simulink model "Target_Control_System"  (R2021b)
settings: Solver=FixedStepDiscrete  StartTime=0.0  StopTime=5  RelTol=1e-3
PreLoadFcn:
  | RTWConfigurationCB('preloadfcn', bdroot);
PostLoadFcn:
  | load('configuration/data_struct.mat');
  | load('configuration/fluxMaps_propMotor.mat');
  | load('configuration/parameterInit_PROP.mat');
  | load('configuration/parameterInit_PUMP.mat');
  | load('configuration/parameterInit_PITCH.mat');
  | load('configuration/parameterInit_TILT.mat');
  | %load('configuration/base_workspace_signal_definition.mat');
  | %load('resolvedatastores_to_baseworkspace_for_faster_simulation.mat');
model workspace (MAT data in the model file):
  SIMULATION_OPTIONS : Simulink.Parameter (value not decoded)
  TARGET_CODE_GEN : Simulink.Parameter (value not decoded)
  TCS_SAMPLE_FREQ_HZ : Simulink.Parameter (value not decoded)
symbols that are objects in the model workspace (value not decoded): TARGET_CODE_GEN, TCS_SAMPLE_FREQ_HZ
undefined symbols (not defined in the file): A_DQ_REF_LPF_INIT__PITCH, A_DQ_REF_LPF_INIT__PROP, A_DQ_REF_LPF_INIT__PUMP, A_DQ_REF_LPF_INIT__TILT, A_OBSERVER_CONFIDENCE_INIT__PITCH, A_OBSERVER_CONFIDENCE_INIT__PROP, A_OBSERVER_CONFIDENCE_INIT__PUMP, A_OBSERVER_CONFIDENCE_INIT__TILT, ACTUATOR_MAX_ANGLE_TRIP__PITCH, ACTUATOR_MIN_ANGLE_TRIP__PITCH, ACTUATOR_POS_SENSOR_INV_DIRECTION__PITCH, ACTUATOR_POS_SENSOR_INV_DIRECTION__TILT, ACTUATOR_POS_SENSOR_OFFSET__PITCH, ACTUATOR_POS_SENSOR_OFFSET__TILT, ADC_scaler1_baseaddr_TILT, ADC_SCALER_FLOAT_TO_FIXPOINT_EXPANSION, ANGLE_ELEC_FROM_SENSOR_OFFSET_INIT__PITCH, ANGLE_ELEC_FROM_SENSOR_OFFSET_INIT__PROP, ANGLE_ELEC_FROM_SENSOR_OFFSET_INIT__PUMP, ANGLE_ELEC_FROM_SENSOR_OFFSET_INIT__TILT, AUTO_CLEAR_FAULTS_ENABLED__PITCH, AUTO_CLEAR_FAULTS_ENABLED__PROP, AUTO_CLEAR_FAULTS_ENABLED__PUMP, AUTO_CLEAR_FAULTS_ENABLED__TILT, AUTO_CLEAR_FAULTS_WAIT_TICKS__PITCH, AUTO_CLEAR_FAULTS_WAIT_TICKS__PROP, AUTO_CLEAR_FAULTS_WAIT_TICKS__PUMP, AUTO_CLEAR_FAULTS_WAIT_TICKS__TILT, AUTO_I_ZERO_IDLE_TICKS__PITCH, AUTO_I_ZERO_IDLE_TICKS__PROP, AUTO_I_ZERO_IDLE_TICKS__PUMP, AUTO_I_ZERO_IDLE_TICKS__TILT, AUTO_I_ZERO_OFFSET_IDC_THRESHOLD__PITCH, AUTO_I_ZERO_OFFSET_IDC_THRESHOLD__PROP, AUTO_I_ZERO_OFFSET_IDC_THRESHOLD__PUMP, AUTO_I_ZERO_OFFSET_IDC_THRESHOLD__TILT, AUTO_I_ZERO_OFFSET_IPH_THRESHOLD__PITCH, AUTO_I_ZERO_OFFSET_IPH_THRESHOLD__PROP, AUTO_I_ZERO_OFFSET_IPH_THRESHOLD__PUMP, AUTO_I_ZERO_OFFSET_IPH_THRESHOLD__TILT, AUTO_SENSORLESS_SWITCHOVER_DISABLE_OMEGA, AUTO_SENSORLESS_SWITCHOVER_ENABLE_OMEGA, AUTO_SENSORLESS_SWITCHOVER_MIN_CONFIDENCE, AUXILIARY_PROTECTION_UNIT_BASEADDR__TILT, blanking_max_error_omega_INIT_PITCH, blanking_max_error_omega_INIT_TILT, blanking_max_error_position_INIT_PITCH, blanking_max_error_position_INIT_TILT, BRUTE_START_I_Q_REF_RAMP_SPEED__PITCH, BRUTE_START_I_Q_REF_RAMP_SPEED__PROP, BRUTE_START_I_Q_REF_RAMP_SPEED__PUMP, BRUTE_START_I_Q_REF_RAMP_SPEED__TILT, CONTROL_LOOP_DT_INIT__PITCH, CONTROL_LOOP_DT_INIT__PROP, CONTROL_LOOP_DT_INIT__PUMP, CONTROL_LOOP_DT_INIT__TILT, CORRECTION_FILTER_SCALE__PITCH, CORRECTION_FILTER_SCALE__PROP, CORRECTION_FILTER_SCALE__PUMP, CORRECTION_FILTER_SCALE__TILT ... (+458)
libraries: simulink x178, Reusables_Lib x24
(part 6 of 47)

== system Target_Control_System/Target_Control_System/InterruptFunction/pitchMotor_isrTask/abcToAlphaBeta ==
  abcToAlphaBeta : TriggerPort  TriggerType=function-call  VariantControl=Variant
  Alpha-Beta Calcs1 : Subsystem
  Calc Angle From Speed : Subsystem
  Constant1 : Constant  Value=TARGET_CODE_GEN  SampleTime=-1
  Data Store Read1 : DataStoreRead  DataStoreName=oPitch  DataStoreElements=oPitch.oIsr_.oState_.fUbPostlpf_  IndexOptions=Index vector (dialog)  Indices=1  OutputSizes=1
  Data Store Read13 : DataStoreRead  DataStoreName=oPitch  DataStoreElements=oPitch.oIsr_.oIn_.oAdcData_.fIa_  IndexOptions=Index vector (dialog)  Indices=1  OutputSizes=1
  Data Store Read14 : DataStoreRead  DataStoreName=oPitch  DataStoreElements=oPitch.oIsr_.oIn_.oAdcData_.fIb_  IndexOptions=Index vector (dialog)  Indices=1  OutputSizes=1
  Data Store Read15 : DataStoreRead  DataStoreName=oPitch  DataStoreElements=oPitch.oIsr_.oIn_.oAdcData_.fIc_  IndexOptions=Index vector (dialog)  Indices=1  OutputSizes=1
  Data Store Read16 : DataStoreRead  DataStoreName=oPitch  DataStoreElements=oPitch.oIsr_.oState_.fUaPostlpf_  IndexOptions=Index vector (dialog)  Indices=1  OutputSizes=1
  Data Store Read17 : DataStoreRead  DataStoreName=oPitch  DataStoreElements=oPitch.oIsr_.oState_.fUcPostlpf_  IndexOptions=Index vector (dialog)  Indices=1  OutputSizes=1
  Data Store Read2 : DataStoreRead  DataStoreName=oPitch  DataStoreElements=oPitch.oIsr_.oIn_.fUphFilterDelayAngleRad_  IndexOptions=Index vector (dialog)  Indices=1  OutputSizes=1
  Data Store Read4 : DataStoreRead  DataStoreName=oPitch  DataStoreElements=oPitch.oIsr_.oState_.fOmegaEObserverRaw2_  IndexOptions=Index vector (dialog)  Indices=1  OutputSizes=1
  Data Store Read8 : DataStoreRead  DataStoreName=oPitch  DataStoreElements=oPitch.oIsr_.oParam_.iInverseDirection_  IndexOptions=Index vector (dialog)  Indices=1  OutputSizes=1
  Data Store Write1 : DataStoreWrite  DataStoreName=oPitch  DataStoreElements=oPitch.oIsr_.oState_.fFluxMainAngleUltraRaw_  IndexOptions=Index vector (dialog)  Indices=1  OutputSizes=1
  Data Store Write2 : DataStoreWrite  DataStoreName=oPitch  DataStoreElements=oPitch.oIsr_.oState_.fIAlpha_  IndexOptions=Index vector (dialog)  Indices=1  OutputSizes=1
  Data Store Write3 : DataStoreWrite  DataStoreName=oPitch  DataStoreElements=oPitch.oIsr_.oState_.fIBeta_  IndexOptions=Index vector (dialog)  Indices=1  OutputSizes=1
  Data Store Write4 : DataStoreWrite  DataStoreName=oPitch  DataStoreElements=oPitch.oIsr_.oState_.fUAlpha_  IndexOptions=Index vector (dialog)  Indices=1  OutputSizes=1
  Data Store Write5 : DataStoreWrite  DataStoreName=oPitch  DataStoreElements=oPitch.oIsr_.oState_.fUBeta_  IndexOptions=Index vector (dialog)  Indices=1  OutputSizes=1
  ModelSource : Subsystem  Commented=on  Variant=on
  NOT1 : Logic  Operator=NOT  AllPortsSameDT=off  OutDataTypeStr=boolean
  vsincos()1 : Subsystem  TreatAsAtomicUnit=on
  wires:
  Data Store Read4/1 -> Calc Angle From Speed/1(Omega)
  NOT1/1 -> vsincos()1/Enable
  Alpha-Beta Calcs1/1(fIAlpha) -> Data Store Write2/1
  Data Store Read16/1 -> Alpha-Beta Calcs1/5(fUaPostlpf)
  Data Store Read8/1 -> Alpha-Beta Calcs1/1(iInverseDirection)
  Data Store Read1/1 -> Alpha-Beta Calcs1/6(fUbPostlpf)
  Alpha-Beta Calcs1/3(fUAlpha) -> Data Store Write4/1
  Data Store Read15/1 -> Alpha-Beta Calcs1/4(fIc)
  Alpha-Beta Calcs1/2(fIBeta) -> Data Store Write3/1
  Constant1/1 -> NOT1/1
  Data Store Read13/1 -> Alpha-Beta Calcs1/2(fIa)
  Data Store Read17/1 -> Alpha-Beta Calcs1/7(fUcPostlpf)
  Data Store Read14/1 -> Alpha-Beta Calcs1/3(fIb)
  Alpha-Beta Calcs1/4(fUBeta) -> Data Store Write5/1
  Calc Angle From Speed/1(fFluxMainAngleRaw2) -> vsincos()1/2(fFluxMainAngleRaw2), Data Store Write1/1
  Data Store Read2/1 -> vsincos()1/1(fUphFilterDelayAngleRad)

== system Target_Control_System/Target_Control_System/InterruptFunction/pitchMotor_isrTask/currentController ==
  currentController : TriggerPort  TriggerType=function-call  VariantControl=Variant
  Current Controller : Subsystem
  Data Store Read4 : DataStoreRead  DataStoreName=oPitch  DataStoreElements=oPitch.oIsr_.oIn_.uiCurrentControllerActive_  IndexOptions=Index vector (dialog)  Indices=1  OutputSizes=1
  wires:
  Data Store Read4/1 -> Current Controller/Enable

== system Target_Control_System/Target_Control_System/InterruptFunction/pitchMotor_isrTask/dqTransform ==
  dqTransform : TriggerPort  TriggerType=function-call  VariantControl=Variant
  DQ Transform : Subsystem
  Data Store Read1 : DataStoreRead  DataStoreName=oPitch  DataStoreElements=oPitch.oIsr_.oState_.fFluxMainMagnitudeLpf_  IndexOptions=Index vector (dialog)  Indices=1  OutputSizes=1
  Data Store Read2 : DataStoreRead  DataStoreName=oPitch  DataStoreElements=oPitch.oIsr_.oState_.fIBeta_  IndexOptions=Index vector (dialog)  Indices=1  OutputSizes=1
  Data Store Read3 : DataStoreRead  DataStoreName=oPitch  DataStoreElements=oPitch.oIsr_.oState_.fIq_  IndexOptions=Index vector (dialog)  Indices=1  OutputSizes=1
  Data Store Read4 : DataStoreRead  DataStoreName=oPitch  DataStoreElements=oPitch.oMot_.oParam_.fPolePairs_  IndexOptions=Index vector (dialog)  Indices=1  OutputSizes=1
  Data Store Read5 : DataStoreRead  DataStoreName=oPitch  DataStoreElements=oPitch.oIsr_.oState_.fIAlpha_  IndexOptions=Index vector (dialog)  Indices=1  OutputSizes=1
  Data Store Write1 : DataStoreWrite  DataStoreName=oPitch  DataStoreElements=oPitch.oIsr_.oOut_.fTEstimate_  IndexOptions=Index vector (dialog)  Indices=1  OutputSizes=1
  Data Store Write2 : DataStoreWrite  DataStoreName=oPitch  DataStoreElements=oPitch.oIsr_.oState_.fId_  IndexOptions=Index vector (dialog)  Indices=1  OutputSizes=1
  Data Store Write3 : DataStoreWrite  DataStoreName=oPitch  DataStoreElements=oPitch.oIsr_.oState_.fIq_  IndexOptions=Index vector (dialog)  Indices=1  OutputSizes=1
  Data Store Write4 : DataStoreWrite  DataStoreName=oPitch  DataStoreElements=oPitch.oIsr_.oOut_.fIPhaseMagnitude_  IndexOptions=Index vector (dialog)  Indices=1  OutputSizes=1
  Torque_Estimation_Pitch : Subsystem
  wires:
  DQ Transform/1(fId) -> Data Store Write2/1
  DQ Transform/3(fIPhaseMagnitude) -> Data Store Write4/1
  Data Store Read3/1 -> Torque_Estimation_Pitch/3(fIq)
  Torque_Estimation_Pitch/1(fTEstimate) -> Data Store Write1/1
  Data Store Read5/1 -> DQ Transform/1(fIAlpha)
  Data Store Read1/1 -> Torque_Estimation_Pitch/2(fFluxMainMagnitudeLpf)
  Data Store Read2/1 -> DQ Transform/2(fIBeta)
  Data Store Read4/1 -> Torque_Estimation_Pitch/1(fPolePairs)
  DQ Transform/2(fIq) -> Data Store Write3/1

== system Target_Control_System/Target_Control_System/InterruptFunction/pitchMotor_isrTask/fluxAngleCalculations ==
  fluxAngleCalculation : TriggerPort  TriggerType=function-call  VariantControl=Variant
  Advance Forced Angle : Subsystem
  Back Rotation : Subsystem
  Constant5 : Constant  Value=TARGET_CODE_GEN  SampleTime=-1
  Data Store Read10 : DataStoreRead  DataStoreName=oPitch  DataStoreElements=oPitch.oIsr_.oIn_.uiForcedAngle_  IndexOptions=Index vector (dialog)  Indices=1  OutputSizes=1
  Data Store Read2 : DataStoreRead  DataStoreName=oPitch  DataStoreElements=oPitch.oIsr_.oIn_.fOmegaERefRampOut_  IndexOptions=Index vector (dialog)  Indices=1  OutputSizes=1
  Data Store Read3 : DataStoreRead  DataStoreName=oPitch  DataStoreElements=oPitch.oIsr_.oParam_.iUseSensorAngle_  IndexOptions=Index vector (dialog)  Indices=1  OutputSizes=1
  Data Store Read4 : DataStoreRead  DataStoreName=oPitch  DataStoreElements=oPitch.oIsr_.oIn_.fFluxMasterAngleForced2closedSmoothingRampOut_  IndexOptions=Index vector (dialog)  Indices=1  OutputSizes=1
  Data Store Read5 : DataStoreRead  DataStoreName=oPitch  DataStoreElements=oPitch.oIsr_.oIn_.fOmegaElecFromPosSensor_  IndexOptions=Index vector (dialog)  Indices=1  OutputSizes=1
  Data Store Read6 : DataStoreRead  DataStoreName=oPitch  DataStoreElements=oPitch.oIsr_.oIn_.fFluxMasterAngleOffsetRampOut_  IndexOptions=Index vector (dialog)  Indices=1  OutputSizes=1
  Data Store Read7 : DataStoreRead  DataStoreName=oPitch  DataStoreElements=oPitch.oIsr_.oState_.fOmegaEObserverLpf2_  IndexOptions=Index vector (dialog)  Indices=1  OutputSizes=1
  Data Store Read8 : DataStoreRead  DataStoreName=oPitch  DataStoreElements=oPitch.oIsr_.oIn_.fAngleElecFromPosSensor_  IndexOptions=Index vector (dialog)  Indices=1  OutputSizes=1
  Data Store Read9 : DataStoreRead  DataStoreName=oPitch  DataStoreElements=oPitch.oIsr_.oState_.fFluxMainAngleRaw2_  IndexOptions=Index vector (dialog)  Indices=1  OutputSizes=1
  Data Store Write21 : DataStoreWrite  DataStoreName=mdl_pitch_fOmegaE  IndexOptions=Index vector (dialog)  Indices=1  OutputSizes=1
  Data Store Write3 : DataStoreWrite  DataStoreName=oPitch  DataStoreElements=oPitch.oIsr_.oState_.fFluxMasterAngleBkwd_  IndexOptions=Index vector (dialog)  Indices=1  OutputSizes=1
  Data Store Write4 : DataStoreWrite  DataStoreName=oPitch  DataStoreElements=oPitch.oIsr_.oState_.fFluxMasterAngle_  IndexOptions=Index vector (dialog)  Indices=1  OutputSizes=1
  Equal4 : RelationalOperator  Operator===  OutDataTypeStr=boolean  RndMeth=Simplest
  ModelSource : Subsystem  Variant=on
  NOT2 : Logic  Operator=NOT  AllPortsSameDT=off  OutDataTypeStr=boolean
  Not forced Angle : Subsystem
  One3 : Constant  OutDataTypeStr=uint32  SampleTime=-1
  Switch1 : Switch  Criteria=u2 > Threshold  Threshold=0.5
  Switch2 : Switch  Criteria=u2 > Threshold  Threshold=0.5
  vsincos() : Subsystem  TreatAsAtomicUnit=on
  wires:
  Advance Forced Angle/1(Output) -> Switch2/1
  Data Store Read7/1 -> Not forced Angle/5(fOmegaEObserverLpf2)
  Data Store Read6/1 -> Back Rotation/1(fFluxMasterAngleOffsetRampOut)
  Data Store Read5/1 -> Not forced Angle/4(fOmegaElecFromPosSensor)
  Data Store Read4/1 -> Not forced Angle/6(fFluxMasterAngleForced2closedSmoothingRampOut)
  Equal4/1 -> Switch1/2, Switch2/2
  Constant5/1 -> NOT2/1
  Not forced Angle/1(fFluxMasterAngle) -> Switch2/3
  Data Store Read8/1 -> Not forced Angle/2(fAngleElecFromPosSensor)
  Data Store Read3/1 -> Not forced Angle/1(iUseSensorAngle)
  Switch1/1 -> Data Store Write21/1
  Data Store Read2/1 -> Advance Forced Angle/1(Input), Switch1/1
  One3/1 -> Equal4/2
  NOT2/1 -> vsincos()/Enable
  Not forced Angle/2(fOmegaE) -> Switch1/3
  Data Store Read10/1 -> Equal4/1
  Back Rotation/1(fFluxMasterAngleBkwd) -> Data Store Write3/1, vsincos()/1(fFluxMasterAngleBkwd)
  Data Store Read9/1 -> Not forced Angle/3(fFluxMainAngleRaw2)
  Switch2/1 -> Data Store Write4/1, Back Rotation/2(fFluxMasterAngle), vsincos()/2(fFluxMasterAngle)

== system Target_Control_System/Target_Control_System/InterruptFunction/pitchMotor_isrTask/fluxObserver ==
  fluxObserver : TriggerPort  TriggerType=function-call  VariantControl=Variant
  Calculate Coil Flux + Bleeder : Subsystem
  Calculate Main Flux + LPF : Subsystem
  Data Store Read : DataStoreRead  DataStoreName=oPitch  DataStoreElements=oPitch.oIsr_.oParam_.fRsPhase_  IndexOptions=Index vector (dialog)  Indices=1  OutputSizes=1
  Data Store Read1 : DataStoreRead  DataStoreName=oPitch  DataStoreElements=oPitch.oIsr_.oIn_.fUphFilterAmplitudeRatio_  IndexOptions=Index vector (dialog)  Indices=1  OutputSizes=1
  Data Store Read10 : DataStoreRead  DataStoreName=oPitch  DataStoreElements=oPitch.oIsr_.oParam_.fLsPhase_  IndexOptions=Index vector (dialog)  Indices=1  OutputSizes=1
  Data Store Read11 : DataStoreRead  DataStoreName=oPitch  DataStoreElements=oPitch.oMot_.oParam_.fObserverLoopFilterBandwidthHz_  IndexOptions=Index vector (dialog)  Indices=1  OutputSizes=1
  Data Store Read12 : DataStoreRead  DataStoreName=oPitch  DataStoreElements=oPitch.oIsr_.oParam_.oPiDataPll2_.fState_  IndexOptions=Index vector (dialog)  Indices=1  OutputSizes=1
  Data Store Read13 : DataStoreRead  DataStoreName=oPitch  DataStoreElements=oPitch.oIsr_.oParam_.oPiDataPll2_.oParameter_.fKp_  IndexOptions=Index vector (dialog)  Indices=1  OutputSizes=1
  Data Store Read14 : DataStoreRead  DataStoreName=oPitch  DataStoreElements=oPitch.oIsr_.oParam_.oPiDataPll2_.oParameter_.fKi_  IndexOptions=Index vector (dialog)  Indices=1  OutputSizes=1
  Data Store Read15 : DataStoreRead  DataStoreName=oPitch  DataStoreElements=oPitch.oIsr_.oParam_.oPiDataPll2_.oParameter_.fLoopDt_  IndexOptions=Index vector (dialog)  Indices=1  OutputSizes=1
  Data Store Read16 : DataStoreRead  DataStoreName=oPitch  DataStoreElements=oPitch.oIsr_.oParam_.oPiDataPll2_.oParameter_.fIntMax_  IndexOptions=Index vector (dialog)  Indices=1  OutputSizes=1
  Data Store Read17 : DataStoreRead  DataStoreName=oPitch  DataStoreElements=oPitch.oIsr_.oParam_.oPiDataPll2_.oParameter_.fOutMax_  IndexOptions=Index vector (dialog)  Indices=1  OutputSizes=1
  Data Store Read18 : DataStoreRead  DataStoreName=oPitch  DataStoreElements=oPitch.oIsr_.oParam_.oPiDataPll2_.oParameter_.fIntMin_  IndexOptions=Index vector (dialog)  Indices=1  OutputSizes=1
  Data Store Read19 : DataStoreRead  DataStoreName=oPitch  DataStoreElements=oPitch.oIsr_.oParam_.oPiDataPll2_.oParameter_.fOutMin_  IndexOptions=Index vector (dialog)  Indices=1  OutputSizes=1
  Data Store Read2 : DataStoreRead  DataStoreName=mdl_pitch_fFluxMainAngleRaw2_sin_  IndexOptions=Index vector (dialog)  Indices=1  OutputSizes=1
  Data Store Read27 : DataStoreRead  DataStoreName=mdl_pitch_fUphFilterDelayAngleRad_sin_  IndexOptions=Index vector (dialog)  Indices=1  OutputSizes=1
  Data Store Read28 : DataStoreRead  DataStoreName=mdl_pitch_fUphFilterDelayAngleRad_cos_  IndexOptions=Index vector (dialog)  Indices=1  OutputSizes=1
  Data Store Read3 : DataStoreRead  DataStoreName=oPitch  DataStoreElements=oPitch.oIsr_.oParam_.uiUphFilterCorrectionEnabled_  IndexOptions=Index vector (dialog)  Indices=1  OutputSizes=1
  Data Store Read34 : DataStoreRead  DataStoreName=mdl_pitch_fFluxMainAngleRaw2_cos_  IndexOptions=Index vector (dialog)  Indices=1  OutputSizes=1
  Data Store Read4 : DataStoreRead  DataStoreName=oPitch  DataStoreElements=oPitch.oIsr_.oState_.fUAlpha_  IndexOptions=Index vector (dialog)  Indices=1  OutputSizes=1
  Data Store Read5 : DataStoreRead  DataStoreName=oPitch  DataStoreElements=oPitch.oIsr_.oState_.fUBeta_  IndexOptions=Index vector (dialog)  Indices=1  OutputSizes=1
  Data Store Read6 : DataStoreRead  DataStoreName=oPitch  DataStoreElements=oPitch.oIsr_.oState_.fIAlpha_  IndexOptions=Index vector (dialog)  Indices=1  OutputSizes=1
  Data Store Read7 : DataStoreRead  DataStoreName=oPitch  DataStoreElements=oPitch.oIsr_.oState_.fIBeta_  IndexOptions=Index vector (dialog)  Indices=1  OutputSizes=1
  Data Store Read8 : DataStoreRead  DataStoreName=oPitch  DataStoreElements=oPitch.oIsr_.oParam_.fControlLoopDt_  IndexOptions=Index vector (dialog)  Indices=1  OutputSizes=1
  Data Store Read9 : DataStoreRead  DataStoreName=oPitch  DataStoreElements=oPitch.oIsr_.oParam_.fKFluxBleeder_  IndexOptions=Index vector (dialog)  Indices=1  OutputSizes=1
  Data Store Write1 : DataStoreWrite  DataStoreName=oPitch  DataStoreElements=oPitch.oIsr_.oState_.fFluxCoilAlpha_  IndexOptions=Index vector (dialog)  Indices=1  OutputSizes=1
  Data Store Write10 : DataStoreWrite  DataStoreName=oPitch  DataStoreElements=oPitch.oIsr_.oState_.fAtan2loopfilter2Out_  IndexOptions=Index vector (dialog)  Indices=1  OutputSizes=1
  Data Store Write11 : DataStoreWrite  DataStoreName=oPitch  DataStoreElements=oPitch.oIsr_.oParam_.oPiDataPll2_.fState_  IndexOptions=Index vector (dialog)  Indices=1  OutputSizes=1
  Data Store Write12 : DataStoreWrite  DataStoreName=oPitch  DataStoreElements=oPitch.oIsr_.oState_.fOmegaEObserverRaw2_  IndexOptions=Index vector (dialog)  Indices=1  OutputSizes=1
  Data Store Write13 : DataStoreWrite  DataStoreName=oPitch  DataStoreElements=oPitch.oIsr_.oState_.fOmegaEObserverLpf2_  IndexOptions=Index vector (dialog)  Indices=1  OutputSizes=1
  Data Store Write14 : DataStoreWrite  DataStoreName=oPitch  DataStoreElements=oPitch.oIsr_.oState_.fFluxMainMagnitudeLpf_  IndexOptions=Index vector (dialog)  Indices=1  OutputSizes=1
  Data Store Write15 : DataStoreWrite  DataStoreName=oPitch  DataStoreElements=oPitch.oIsr_.oState_.fFluxMainMagnitude_  IndexOptions=Index vector (dialog)  Indices=1  OutputSizes=1
  Data Store Write2 : DataStoreWrite  DataStoreName=oPitch  DataStoreElements=oPitch.oIsr_.oState_.fUBeta_  IndexOptions=Index vector (dialog)  Indices=1  OutputSizes=1
  Data Store Write28 : DataStoreWrite  DataStoreName=oPitch  DataStoreElements=oPitch.oIsr_.oState_.fIAlphaLpf4hpf_  IndexOptions=Index vector (dialog)  Indices=1  OutputSizes=1
  Data Store Write29 : DataStoreWrite  DataStoreName=oPitch  DataStoreElements=oPitch.oIsr_.oState_.fIBetaLpf4hpf_  IndexOptions=Index vector (dialog)  Indices=1  OutputSizes=1
  Data Store Write3 : DataStoreWrite  DataStoreName=oPitch  DataStoreElements=oPitch.oIsr_.oState_.fUAlphaLpf4hpf_  IndexOptions=Index vector (dialog)  Indices=1  OutputSizes=1
  Data Store Write4 : DataStoreWrite  DataStoreName=oPitch  DataStoreElements=oPitch.oIsr_.oState_.fUBetaLpf4hpf_  IndexOptions=Index vector (dialog)  Indices=1  OutputSizes=1
  Data Store Write5 : DataStoreWrite  DataStoreName=oPitch  DataStoreElements=oPitch.oIsr_.oState_.fUAlpha_  IndexOptions=Index vector (dialog)  Indices=1  OutputSizes=1
  Data Store Write6 : DataStoreWrite  DataStoreName=oPitch  DataStoreElements=oPitch.oIsr_.oState_.fFluxCoilBeta_  IndexOptions=Index vector (dialog)  Indices=1  OutputSizes=1
  Data Store Write7 : DataStoreWrite  DataStoreName=oPitch  DataStoreElements=oPitch.oIsr_.oState_.fFluxMainAlpha_  IndexOptions=Index vector (dialog)  Indices=1  OutputSizes=1
  Data Store Write8 : DataStoreWrite  DataStoreName=oPitch  DataStoreElements=oPitch.oIsr_.oState_.fFluxMainBeta_  IndexOptions=Index vector (dialog)  Indices=1  OutputSizes=1
  Data Store Write9 : DataStoreWrite  DataStoreName=oPitch  DataStoreElements=oPitch.oIsr_.oState_.fFluxMainAngleUltraRaw_  IndexOptions=Index vector (dialog)  Indices=1  OutputSizes=1
  Fast PLL : Subsystem
  HPF Currents : Subsystem
  HPF Voltages : Subsystem
  Mux : Mux  Inputs=7
  Subtract Resistive Voltage Drop : Subsystem
  Ultra Raw Angle : Subsystem
  Voltage Vector Rotation : Subsystem
  wires:
  Data Store Read34/1 -> Fast PLL/2(fluxAngle_cos)
  Data Store Read19/1 -> Mux/7
  Data Store Read1/1 -> Voltage Vector Rotation/3(fUphFilterAmplitudeRatio)
  HPF Currents/2(fIBetaLpf4hpf) -> Data Store Write29/1
  Calculate Main Flux + LPF/4(fFluxMainMagnitudeLpf) -> Data Store Write14/1
  Calculate Main Flux + LPF/3(fFluxMainMagnitude) -> Data Store Write15/1
  Data Store Read/1 -> Subtract Resistive Voltage Drop/3(fRsPhase)
  Data Store Read27/1 -> Voltage Vector Rotation/1(UphFilterDelayAngleRad_sin)
  Data Store Read17/1 -> Mux/5
  Data Store Read18/1 -> Mux/6
  Data Store Read2/1 -> Fast PLL/1(fluxAngle_sin)
  Data Store Read9/1 -> Calculate Coil Flux + Bleeder/2(fKFluxBleeder)
  HPF Currents/3(fIAlphaLocal) -> Calculate Main Flux + LPF/1(fIAlphaLocal), Subtract Resistive Voltage Drop/1(fIAlphaLocal)  "fIAlphaLocal"
  Data Store Read15/1 -> Mux/3
  HPF Voltages/3(fUAlpha_out) -> Data Store Write5/1, Calculate Coil Flux + Bleeder/3(fUAlpha)
  Data Store Read14/1 -> Mux/2
  Data Store Read13/1 -> Mux/1
  Calculate Coil Flux + Bleeder/2(fFluxCoilBeta) -> Calculate Main Flux + LPF/5(fFluxCoilBeta), Data Store Write6/1
  Calculate Coil Flux + Bleeder/1(fFluxCoilAlpha) -> Calculate Main Flux + LPF/4(fFluxCoilAlpha), Data Store Write1/1
  Data Store Read4/1 -> Voltage Vector Rotation/5(fUAlpha)
  Calculate Main Flux + LPF/1(fFluxMainAlpha) -> Data Store Write7/1, Fast PLL/3(fFluxMainAlpha), Ultra Raw Angle/1(fFluxMainAlpha)
  Fast PLL/4(fOmegaEObserverLpf2) -> Data Store Write13/1
  HPF Voltages/4(fUBeta_out) -> Calculate Coil Flux + Bleeder/4(fUBeta), Data Store Write2/1
  HPF Currents/1(fIAlphaLpf4hpf) -> Data Store Write28/1
  Data Store Read3/1 -> Voltage Vector Rotation/4(uiUphFilterCorrectionEnabled)
  Data Store Read7/1 -> HPF Currents/2(fIBeta)
  HPF Currents/4(fIBetaLocal) -> Calculate Main Flux + LPF/2(fIBetaLocal), Subtract Resistive Voltage Drop/2(fIBetaLocal)  "fIBetaLocal"
  Subtract Resistive Voltage Drop/1(fUAlpha_out) -> HPF Voltages/1(fUAlpha)
  HPF Voltages/1(fUAlphaLpf4hpf) -> Data Store Write3/1
  Data Store Read5/1 -> Voltage Vector Rotation/6(fUBeta)
  Data Store Read16/1 -> Mux/4
  Subtract Resistive Voltage Drop/2(fUBeta_out) -> HPF Voltages/2(fUBeta)
  Data Store Read10/1 -> Calculate Main Flux + LPF/3(fLsPhase)
  Voltage Vector Rotation/2(fUBeta_out) -> Subtract Resistive Voltage Drop/5(fUBeta)
  Calculate Main Flux + LPF/2(fFluxMainBeta) -> Fast PLL/4(fFluxMainBeta), Ultra Raw Angle/2(fFluxMainBeta), Data Store Write8/1
  HPF Voltages/2(fUBetaLpf4hpf) -> Data Store Write4/1
  Voltage Vector Rotation/1(fUAlpha_out) -> Subtract Resistive Voltage Drop/4(fUAlpha)
  Data Store Read8/1 -> Calculate Coil Flux + Bleeder/1(fControlLoopDt)
  Data Store Read28/1 -> Voltage Vector Rotation/2(UphFilterDelayAngleRad_cos)
  Fast PLL/2(oPiDataPll2_.fState*) -> Data Store Write11/1
  Ultra Raw Angle/1(fFluxMainAngleUltraRaw) -> Data Store Write9/1
  Mux/1 -> Fast PLL/7(oPiDataPll2_.oParameter)
  Fast PLL/1(fAtan2loopfilter2Out) -> Data Store Write10/1
  Data Store Read6/1 -> HPF Currents/1(fIAlpha)
  Data Store Read11/1 -> Fast PLL/5(fObserverLoopFilterBandwidthHz)
  Data Store Read12/1 -> Fast PLL/6(oPiDataPll2_.fState)
  Fast PLL/3(fOmegaEObserverRaw2) -> Data Store Write12/1

== system Target_Control_System/Target_Control_System/InterruptFunction/pitchMotor_isrTask/isrStateMachine ==
  isrStateMachine : TriggerPort  TriggerType=function-call  VariantControl=Variant
  ISR State Machine : Stateflow chart  TreatAsAtomicUnit=on

== system Target_Control_System/Target_Control_System/InterruptFunction/pitchMotor_isrTask/pwmGeneration ==
  pwmGeneration : TriggerPort  TriggerType=function-call  VariantControl=Variant
  Data Store Read1 : DataStoreRead  DataStoreName=oPitch  DataStoreElements=oPitch.oIsr_.oIn_.uiCurrentControllerActive_  IndexOptions=Index vector (dialog)  Indices=1  OutputSizes=1
  Subsystem : Subsystem
  wires:
  Data Store Read1/1 -> Subsystem/Enable

== system Target_Control_System/Target_Control_System/InterruptFunction/pitchMotor_isrTask/resetFlags ==
  resetFlags : TriggerPort  TriggerType=function-call  VariantControl=Variant
  Constant1 : Constant  Value=0  OutDataTypeStr=int32  SampleTime=-1
  Data Store Write1 : DataStoreWrite  DataStoreName=oPitch  DataStoreElements=oPitch.oIsr_.oState_.iPwmUpdated_  IndexOptions=Index vector (dialog)  Indices=1  OutputSizes=1
  Data Store Write2 : DataStoreWrite  DataStoreName=oPitch  DataStoreElements=oPitch.oIsr_.oOut_.iIBiasUpdated_  IndexOptions=Index vector (dialog)  Indices=1  OutputSizes=1
  Data Store Write3 : DataStoreWrite  DataStoreName=oPitch  DataStoreElements=oPitch.oIsr_.oOut_.iUBiasUpdated_  IndexOptions=Index vector (dialog)  Indices=1  OutputSizes=1
  wires:
  Constant1/1 -> Data Store Write1/1, Data Store Write2/1, Data Store Write3/1

== system Target_Control_System/Target_Control_System/InterruptFunction/pitchMotor_isrTask/softCurrentLimiting ==
  softCurrentLimiting : TriggerPort  TriggerType=function-call  VariantControl=Variant

== system Target_Control_System/Target_Control_System/InterruptFunction/pitchMotor_setPwm/ModelSourceFPGAPitch ==
  note: 1) Add Subsystem or Model blocks as valid variant choices.
      | 2) You cannot connect blocks at this level. At simulation, connectivity is automatically
      | determined, based on the active variant and port name matching.
  DoNotIncludeCustomCode : Subsystem  TreatAsAtomicUnit=on  VariantControl=TARGET_CODE_GEN == 0
  IncludeCustomCode : Subsystem  TreatAsAtomicUnit=on  VariantControl=(default)

== system Target_Control_System/Target_Control_System/InterruptFunction/pitchMotor_setPwm/Subsystem ==
  note: // signal to the pwm block that we handled the interrupt
  Enable : EnablePort
  Constant10 : Constant  OutDataTypeStr=int32  SampleTime=-1
  Data Store Read2 : DataStoreRead  DataStoreName=oPitch  DataStoreElements=oPitch.oIsr_.oParam_.fPwmPeriodTicksFloat_  IndexOptions=Index vector (dialog)  Indices=1  OutputSizes=1
  Data Store Write : DataStoreWrite  DataStoreName=oPitch  DataStoreElements=oPitch.oIsr_.oOut_.uiPwmDutyTicksA_  IndexOptions=Index vector (dialog)  Indices=1  OutputSizes=1
  Data Type Conversion : DataTypeConversion  OutDataTypeStr=uint32
  Shift Arithmetic1 : ArithShift  BitShiftNumberSource=Input port  BitShiftNumber=8  BitShiftDirection=Right
      settings: InputPortMap=u0,p1
  wires:
  Shift Arithmetic1/1 -> Data Type Conversion/1
  Data Type Conversion/1 -> Data Store Write/1
  Data Store Read2/1 -> Shift Arithmetic1/1
  Constant10/1 -> Shift Arithmetic1/2

== system Target_Control_System/Target_Control_System/InterruptFunction/propMotor_IsrSchedule/Isr_Variant ==
  note: 1) Add Subsystem or Model blocks as valid variant choices.
      | 2) You cannot connect blocks at this level. At simulation, connectivity is automatically
      | determined, based on the active variant and port name matching.
  CodeGen_IsrEnable : Subsystem  VariantControl=false
  Simulation_IsrEnable : Subsystem  VariantControl=true
  IsrCall : Outport

== system Target_Control_System/Target_Control_System/InterruptFunction/propMotor_isrTask/abcToAlphaBeta ==
  abcToAlphaBeta : TriggerPort  TriggerType=function-call  VariantControl=Variant
  Constant1 : Constant  Value=TARGET_CODE_GEN  SampleTime=-1
  Data Store Read10 : DataStoreRead  DataStoreName=oProp  DataStoreElements=oProp.oIsr_.oState_.fUaPostlpf_  IndexOptions=Index vector (dialog)  Indices=1  OutputSizes=1
  Data Store Read11 : DataStoreRead  DataStoreName=oProp  DataStoreElements=oProp.oIsr_.oIn_.oAdcData_.fIb_  IndexOptions=Index vector (dialog)  Indices=1  OutputSizes=1
  Data Store Read12 : DataStoreRead  DataStoreName=oProp  DataStoreElements=oProp.oIsr_.oIn_.oAdcData_.fIc_  IndexOptions=Index vector (dialog)  Indices=1  OutputSizes=1
  Data Store Read18 : DataStoreRead  DataStoreName=oProp  DataStoreElements=oProp.oIsr_.oParam_.iInverseDirection_  IndexOptions=Index vector (dialog)  Indices=1  OutputSizes=1
  Data Store Read3 : DataStoreRead  DataStoreName=oProp  DataStoreElements=oProp.oIsr_.oIn_.fUphFilterDelayAngleRad_  IndexOptions=Index vector (dialog)  Indices=1  OutputSizes=1
  Data Store Read5 : DataStoreRead  DataStoreName=oProp  DataStoreElements=oProp.oIsr_.oParam_.iInverseDirection_  IndexOptions=Index vector (dialog)  Indices=1  OutputSizes=1
  Data Store Read6 : DataStoreRead  DataStoreName=oProp  DataStoreElements=oProp.oIsr_.oState_.fUbPostlpf_  IndexOptions=Index vector (dialog)  Indices=1  OutputSizes=1
  Data Store Read67 : DataStoreRead  DataStoreName=oProp  DataStoreElements=oProp.oIsr_.oState_.fOmegaEObserverRaw2_  IndexOptions=Index vector (dialog)  Indices=1  OutputSizes=1
  Data Store Read7 : DataStoreRead  DataStoreName=oProp  DataStoreElements=oProp.oIsr_.oState_.fUcPostlpf_  IndexOptions=Index vector (dialog)  Indices=1  OutputSizes=1
  Data Store Read9 : DataStoreRead  DataStoreName=oProp  DataStoreElements=oProp.oIsr_.oIn_.oAdcData_.fIa_  IndexOptions=Index vector (dialog)  Indices=1  OutputSizes=1
  Data Store Write12 : DataStoreWrite  DataStoreName=oProp  DataStoreElements=oProp.oIsr_.oState_.fIAlpha_  IndexOptions=Index vector (dialog)  Indices=1  OutputSizes=1
  Data Store Write13 : DataStoreWrite  DataStoreName=oProp  DataStoreElements=oProp.oIsr_.oState_.fIBeta_  IndexOptions=Index vector (dialog)  Indices=1  OutputSizes=1
  Data Store Write14 : DataStoreWrite  DataStoreName=oProp  DataStoreElements=oProp.oIsr_.oState_.fFluxMainAngleRaw2_  IndexOptions=Index vector (dialog)  Indices=1  OutputSizes=1
  Data Store Write20 : DataStoreWrite  DataStoreName=oProp  DataStoreElements=oProp.oIsr_.oState_.fUBeta_  IndexOptions=Index vector (dialog)  Indices=1  OutputSizes=1
  Data Store Write8 : DataStoreWrite  DataStoreName=oProp  DataStoreElements=oProp.oIsr_.oState_.fUAlpha_  IndexOptions=Index vector (dialog)  Indices=1  OutputSizes=1
  Demux1 : Demux  Outputs=2
  Demux2 : Demux  Outputs=2
  Integrator with Angle Wrapper : Subsystem
  ModelSourceFOProp : Subsystem  Variant=on
  Mux1 : Mux  Inputs=3
  Mux3 : Mux  Inputs=3
  NOT : Logic  Operator=NOT  AllPortsSameDT=off  OutDataTypeStr=boolean
  Switch : Switch  Criteria=u2 > Threshold
  Switch1 : Switch  Criteria=u2 > Threshold
  abc to alpha/beta1 : Gain  Gain="2/3*[1 -0.5 -0.5  ; 0 sqrt(3)/2 -sqrt(3)/2 ]"  Multiplication=Matrix(K*u) (u vector)
  abc to alpha/beta4 : Gain  Gain="2/3*[1 -0.5 -0.5  ; 0 sqrt(3)/2 -sqrt(3)/2 ]"  Multiplication=Matrix(K*u) (u vector)
  abc to alpha/beta_inverseDirection : Gain  Gain="2/3*[1 -0.5 -0.5  ; 0 -sqrt(3)/2 sqrt(3)/2 ]"  Multiplication=Matrix(K*u) (u vector)
  abc to alpha/beta_inverseDirection1 : Gain  Gain="2/3*[1 -0.5 -0.5  ; 0 -sqrt(3)/2 sqrt(3)/2 ]"  Multiplication=Matrix(K*u) (u vector)
  vsincos() : Subsystem  TreatAsAtomicUnit=on
  wires:
  Data Store Read6/1 -> Mux3/2
  Data Store Read10/1 -> Mux3/1
  Data Store Read12/1 -> Mux1/3
  Mux3/1 -> abc to alpha/beta_inverseDirection1/1, abc to alpha/beta1/1
  Constant1/1 -> NOT/1
  abc to alpha/beta_inverseDirection/1 -> Switch/1
  Data Store Read5/1 -> Switch/2
  Integrator with Angle Wrapper/1(Angle) -> vsincos()/2(Input1), Data Store Write14/1  "fFluxMainAngleRaw2_"
  Data Store Read9/1 -> Mux1/1
  NOT/1 -> vsincos()/Enable
  abc to alpha/beta_inverseDirection1/1 -> Switch1/1
  abc to alpha/beta1/1 -> Switch1/3
  abc to alpha/beta4/1 -> Switch/3
  Switch/1 -> Demux1/1
  Demux2/2 -> Data Store Write20/1
  Data Store Read7/1 -> Mux3/3
  Data Store Read67/1 -> Integrator with Angle Wrapper/1(Omega)
  Demux2/1 -> Data Store Write8/1
  Switch1/1 -> Demux2/1
  Mux1/1 -> abc to alpha/beta4/1, abc to alpha/beta_inverseDirection/1
  Demux1/2 -> Data Store Write13/1
  Data Store Read3/1 -> vsincos()/1(Input)
  Demux1/1 -> Data Store Write12/1
  Data Store Read18/1 -> Switch1/2
  Data Store Read11/1 -> Mux1/2

== system Target_Control_System/Target_Control_System/InterruptFunction/propMotor_isrTask/currentController ==
  currentController : TriggerPort  TriggerType=function-call  VariantControl=Variant
  Data Store Read9 : DataStoreRead  DataStoreName=oProp  DataStoreElements=oProp.oIsr_.oIn_.uiCurrentControllerActive_  IndexOptions=Index vector (dialog)  Indices=1  OutputSizes=1
  Subsystem : Subsystem
  wires:
  Data Store Read9/1 -> Subsystem/Enable

== system Target_Control_System/Target_Control_System/InterruptFunction/propMotor_isrTask/dqTransform ==
  dqTransform : TriggerPort  TriggerType=function-call  VariantControl=Variant
  Data Store Read13 : DataStoreRead  DataStoreName=mdl_fFluxMasterAngle_cos_  IndexOptions=Index vector (dialog)  Indices=1  OutputSizes=1
  Data Store Read16 : DataStoreRead  DataStoreName=oProp  DataStoreElements=oProp.oIsr_.oState_.fIAlpha_  IndexOptions=Index vector (dialog)  Indices=1  OutputSizes=1
  Data Store Read24 : DataStoreRead  DataStoreName=oProp  DataStoreElements=oProp.oIsr_.oState_.fIq_  IndexOptions=Index vector (dialog)  Indices=1  OutputSizes=1
  Data Store Read3 : DataStoreRead  DataStoreName=mdl_fFluxMasterAngle_sin_  IndexOptions=Index vector (dialog)  Indices=1  OutputSizes=1
  Data Store Read30 : DataStoreRead  DataStoreName=oProp  DataStoreElements=oProp.oIsr_.oState_.fFluxMainMagnitudeLpf_  IndexOptions=Index vector (dialog)  Indices=1  OutputSizes=1
  Data Store Read32 : DataStoreRead  DataStoreName=oProp  DataStoreElements=oProp.oIsr_.oState_.fIBeta_  IndexOptions=Index vector (dialog)  Indices=1  OutputSizes=1
  Data Store Read61 : DataStoreRead  DataStoreName=oProp  DataStoreElements=oProp.oIsr_.oParam_.fPolePairs_  IndexOptions=Index vector (dialog)  Indices=1  OutputSizes=1
  Data Store Write1 : DataStoreWrite  DataStoreName=oProp  DataStoreElements=oProp.oIsr_.oState_.fId_  IndexOptions=Index vector (dialog)  Indices=1  OutputSizes=1
  Data Store Write10 : DataStoreWrite  DataStoreName=oProp  DataStoreElements=oProp.oIsr_.oOut_.fIPhaseMagnitude_  IndexOptions=Index vector (dialog)  Indices=1  OutputSizes=1
  Data Store Write33 : DataStoreWrite  DataStoreName=oProp  DataStoreElements=oProp.oIsr_.oOut_.fTEstimate_  IndexOptions=Index vector (dialog)  Indices=1  OutputSizes=1
  Data Store Write9 : DataStoreWrite  DataStoreName=oProp  DataStoreElements=oProp.oIsr_.oState_.fIq_  IndexOptions=Index vector (dialog)  Indices=1  OutputSizes=1
  Fcn5 : Fcn  Expr=3/2*u(1)*u(2)*u(3)
  Mux2 : Mux  Inputs=2
  Mux5 : Mux
  Mux6 : Mux  Inputs=3
  Square Root Sum : Fcn  Expr=sqrt((u(1)*u(1))+(u(2)*u(2)))
  fId_ = fCosTerm*opState->fIAlpha_ + fSinTerm*opState->fIBeta_1 : Fcn  Expr=u(4)*u(1)+u(3)*u(2)
  fIq_ = fCosTerm*opState->fIBeta_ - fSinTerm*opState->fIAlpha_1 : Fcn  Expr=u(4)*u(2)-u(3)*u(1)
  wires:
  fId_ = fCosTerm*opState->fIAlpha_ + fSinTerm*opState->fIBeta_1/1 -> Mux2/1, Data Store Write1/1
  Data Store Read3/1 -> Mux5/3
  Data Store Read61/1 -> Mux6/1
  Data Store Read30/1 -> Mux6/2
  Data Store Read16/1 -> Mux5/1
  Fcn5/1 -> Data Store Write33/1
  Data Store Read24/1 -> Mux6/3
  Data Store Read13/1 -> Mux5/4
  Mux6/1 -> Fcn5/1
  Mux5/1 -> fId_ = fCosTerm*opState->fIAlpha_ + fSinTerm*opState->fIBeta_1/1, fIq_ = fCosTerm*opState->fIBeta_ - fSinTerm*opState->fIAlpha_1/1
  Square Root Sum/1 -> Data Store Write10/1
  fIq_ = fCosTerm*opState->fIBeta_ - fSinTerm*opState->fIAlpha_1/1 -> Mux2/2, Data Store Write9/1
  Mux2/1 -> Square Root Sum/1
  Data Store Read32/1 -> Mux5/2

== system Target_Control_System/Target_Control_System/InterruptFunction/propMotor_isrTask/fluxAngleCalculation ==
  fluxAngleCalculation : TriggerPort  TriggerType=function-call  VariantControl=Variant
  Add2 : Sum
  Angle Clip : Subsystem
  Constant5 : Constant  Value=TARGET_CODE_GEN  SampleTime=-1
  Data Store Read1 : DataStoreRead  DataStoreName=oProp  DataStoreElements=oProp.oIsr_.oState_.fFluxMainAngleRaw2_  IndexOptions=Index vector (dialog)  Indices=1  OutputSizes=1
  Data Store Read19 : DataStoreRead  DataStoreName=oProp  DataStoreElements=oProp.oIsr_.oState_.fOmegaEObserverLpf2_  IndexOptions=Index vector (dialog)  Indices=1  OutputSizes=1
  Data Store Read21 : DataStoreRead  DataStoreName=oProp  DataStoreElements=oProp.oIsr_.oIn_.uiForcedAngle_  IndexOptions=Index vector (dialog)  Indices=1  OutputSizes=1
  Data Store Read25 : DataStoreRead  DataStoreName=oProp  DataStoreElements=oProp.oIsr_.oIn_.fOmegaERefRampOut_  IndexOptions=Index vector (dialog)  Indices=1  OutputSizes=1
  Data Store Read26 : DataStoreRead  DataStoreName=oProp  DataStoreElements=oProp.oIsr_.oIn_.fFluxMasterAngleOffsetRampOut_  IndexOptions=Index vector (dialog)  Indices=1  OutputSizes=1
  Data Store Read33 : DataStoreRead  DataStoreName=oProp  DataStoreElements=oProp.oIsr_.oIn_.fFluxMasterAngleForced2closedSmoothingRampOut_  IndexOptions=Index vector (dialog)  Indices=1  OutputSizes=1
  Data Store Write1 : DataStoreWrite  DataStoreName=oProp  DataStoreElements=oProp.oIsr_.oState_.fFluxMasterAngle_  IndexOptions=Index vector (dialog)  Indices=1  OutputSizes=1
  Data Store Write2 : DataStoreWrite  DataStoreName=oProp  DataStoreElements=oProp.oIsr_.oState_.fFluxMasterAngleBkwd_  IndexOptions=Index vector (dialog)  Indices=1  OutputSizes=1
  Data Store Write45 : DataStoreWrite  DataStoreName=mdl_prop_fOmegaE  IndexOptions=Index vector (dialog)  Indices=1  OutputSizes=1
  Equal12 : RelationalOperator  Operator===  OutDataTypeStr=boolean  RndMeth=Simplest
  Equal2 : RelationalOperator  Operator=~=  OutDataTypeStr=boolean  RndMeth=Simplest
  ModelSource : Subsystem  Variant=on
  NOT1 : Logic  Operator=NOT  AllPortsSameDT=off  OutDataTypeStr=boolean
  One2 : Constant  OutDataTypeStr=uint32  SampleTime=-1
  Subsystem : Subsystem
  Subsystem1 : Subsystem
  Switch5 : Switch  Criteria=u2 > Threshold  Threshold=0.5
  Switch6 : Switch  Criteria=u2 > Threshold  Threshold=0.5
  Switch7 : Switch  Criteria=u2 > Threshold  Threshold=0.5
  Zero1 : Constant  Value=0  OutDataTypeStr=single  SampleTime=-1
  vsincos()1 : Subsystem  TreatAsAtomicUnit=on
  wires:
  Zero1/1 -> Equal2/2
  Angle Clip/1(Angle_Out) -> vsincos()1/2(fFluxMasterAngleBdwd), Data Store Write2/1
  Switch5/1 -> Switch6/3, Subsystem1/1(In1)
  Switch6/1 -> Add2/1, vsincos()1/1(fFluxMasterAngle), Data Store Write1/1
  Data Store Read21/1 -> Equal12/1
  Data Store Read26/1 -> Add2/2
  Add2/1 -> Angle Clip/1(Angle_In)
  NOT1/1 -> vsincos()1/Enable
  Data Store Read25/1 -> Switch7/1
  Switch7/1 -> Data Store Write45/1  "fFluxMasterAngle_"
  One2/1 -> Equal12/2
  Data Store Read19/1 -> Switch7/3
  Constant5/1 -> NOT1/1
  Equal12/1 -> Switch5/2, Switch7/2, Subsystem/Enable
  Equal2/1 -> Switch6/2, Subsystem1/Enable
  Subsystem1/1(Angle_Out) -> Switch6/1
  Subsystem/1(Angle) -> Switch5/1
  Data Store Read1/1 -> Switch5/3  "fFluxMainAngleRaw2_"
  Data Store Read33/1 -> Subsystem1/2(In2), Equal2/1
